simulink subsystem "ApplFOCSLLowPrio"  (R2024b)
settings: Solver=VariableStepAuto  StartTime=0.0  StopTime=10.0  RelTol=1e-3
undefined symbols (not defined in the file or in its folder): inverter, pmsm, PU_System
libraries: slpidlib x1
settings Model: Creator=The MathWorks, Inc.  LastModifiedBy=snarayan
settings RTWCC: GPUComputeCapability=3.5  LargeConstantGeneration=WriteOnlyDNNConstantsToDataFiles

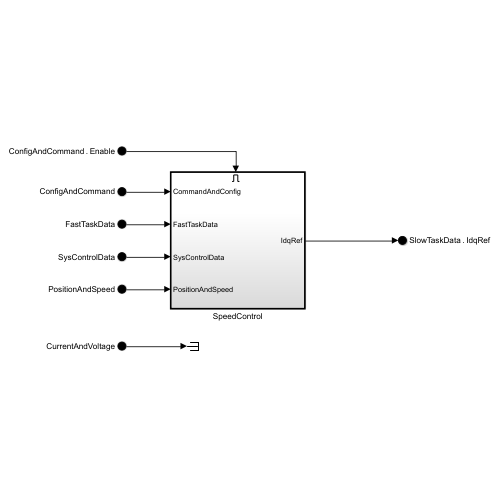
[thumbnail: Simulink's stored preview of the top-level diagram]
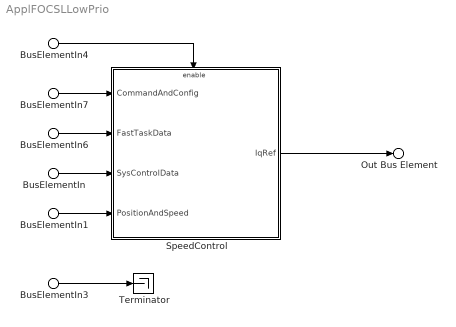
== system ApplFOCSLLowPrio ==
  BusElementIn7 : Inport  PortName=ConfigAndCommand
  BusElementIn4 : Inport  PortName=ConfigAndCommand  Element=Enable
  BusElementIn3 : Inport  Port=2  PortName=CurrentAndVoltage
  BusElementIn1 : Inport  Port=3  PortName=PositionAndSpeed
  BusElementIn6 : Inport  Port=4  PortName=FastTaskData
  BusElementIn : Inport  Port=5  PortName=SysControlData
  SpeedControl : Subsystem
  Terminator : Terminator
  Out Bus Element : Outport  PortName=SlowTaskData  Element=IqRef
  wires:
  BusElementIn4/1 -> SpeedControl/Enable
  SpeedControl/1(IqRef) -> Out Bus Element/1
  BusElementIn7/1 -> SpeedControl/1(CommandAndConfig)
  BusElementIn6/1 -> SpeedControl/2(FastTaskData)
  BusElementIn/1 -> SpeedControl/3(SysControlData)
  BusElementIn1/1 -> SpeedControl/4(PositionAndSpeed)
  BusElementIn3/1 -> Terminator/1

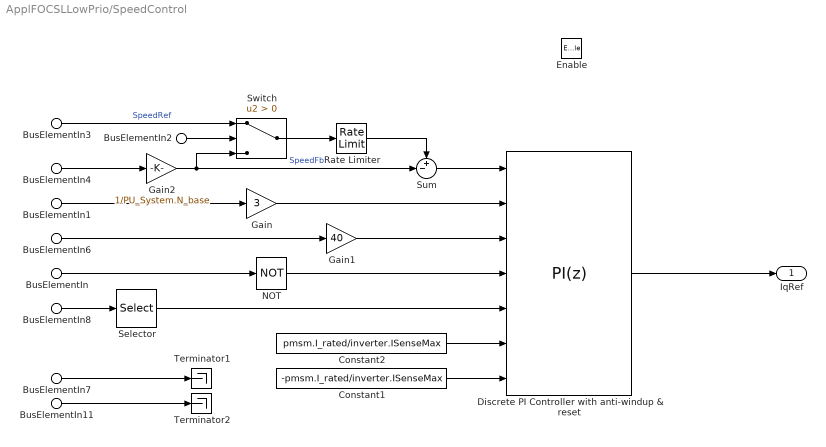
== system ApplFOCSLLowPrio/SpeedControl ==
  BusElementIn11 : Inport  PortName=CommandAndConfig
  BusElementIn : Inport  Port=2  PortName=FastTaskData  Element=EnClosedLoop
  BusElementIn2 : Inport  Port=2  PortName=FastTaskData  Element=EnClosedLoop
  BusElementIn4 : Inport  Port=2  PortName=FastTaskData  Element=Speed
  BusElementIn8 : Inport  Port=2  PortName=FastTaskData  Element=Idq
  BusElementIn1 : Inport  Port=3  PortName=SysControlData  Element=PIGains.Speed_Kp
  BusElementIn6 : Inport  Port=3  PortName=SysControlData  Element=PIGains.Speed_Ki*Tsc
  BusElementIn3 : Inport  Port=3  PortName=SysControlData  Element=SpeedRef
  BusElementIn7 : Inport  Port=4  PortName=PositionAndSpeed
  Enable : EnablePort
  Constant1 : Constant  Value=-pmsm.I_rated/inverter.ISenseMax  OutDataTypeStr=dataType
  Constant2 : Constant  Value=pmsm.I_rated/inverter.ISenseMax  OutDataTypeStr=dataType
  Discrete PI Controller with anti-windup & reset : slpidlib/PID Controller  Controller=PI  Form=Parallel  TimeDomain=Discrete-time  UseExternalTs=off  SampleTime=-1  IntegratorMethod=Forward Euler  FilterMethod=Forward Euler  ControllerParametersSource=external  P=1  I=1  UseKiTs=on  D=0  UseExternalDerivativeSource=off  N=100  UseFilter=on  TunerSelectOption=Transfer Function Based (PID Tuner App)  InitialConditionSource=external  InitialConditionForIntegrator=0  InitialConditionForFilter=0  DifferentiatorICPrevScaledInput=0  ExternalReset=level  TrackingMode=off  Kt=1  LimitOutput=on  SatLimitsSource=external  UpperSaturationLimit=1  LowerSaturationLimit=-1  LinearizeAsGain=on  AntiWindupMode=clamping  Kb=1  LimitIntegrator=off  UpperIntegratorSaturationLimit=inf  LowerIntegratorSaturationLimit=-inf  RndMeth=Simplest  POutMin=[]  POutMax=[]  IOutMin=[]  IOutMax=[]  DOutMin=[]  DOutMax=[]  NOutMin=[]  NOutMax=[]  SumOutMin=[]  SumOutMax=[]  SaturationOutDataTypeStr=Inherit: Inherit via back propagation  SaturationOutMin=[]  SaturationOutMax=[]  PParamMin=[]  PParamMax=[]  IParamMin=[]  IParamMax=[]  DParamMin=[]  DParamMax=[]  NParamMin=[]  NParamMax=[]  KbParamMin=[]  KbParamMax=[]  KtParamMin=[]  KtParamMax=[]  KbOutMin=[]  KbOutMax=[]  KtOutMin=[]  KtOutMax=[]  IntegratorOutMin=[]  IntegratorOutMax=[]  FilterOutMin=[]  FilterOutMax=[]  SumI1OutMin=[]  SumI1OutMax=[]  SumI2OutMin=[]  SumI2OutMax=[]  SumI3OutMin=[]  SumI3OutMax=[]  SumI4OutMin=[]  SumI4OutMax=[]  SumDOutMin=[]  SumDOutMax=[]  DifferentiatorOutMin=[]  DifferentiatorOutMax=[]  FilterDiffOutCoefMin=[]  FilterDiffOutCoefMax=[]  ReciprocalOutMin=[]  ReciprocalOutMax=[]  SumDenOutMin=[]  SumDenOutMax=[]  SumNumOutMin=[]  SumNumOutMax=[]  DivideOutMin=[]  DivideOutMax=[]  UdiffTsProdOutMin=[]  UdiffTsProdOutMax=[]  NTsProdOutMin=[]  NTsProdOutMax=[]  UintegralTsProdOutMin=[]  UintegralTsProdOutMax=[]  UngainTsProdOutMin=[]  UngainTsProdOutMax=[]  ClampingZeroOutDataTypeStr=Inherit: Inherit via back propagation  ClampingZeroOutMin=[]  ClampingZeroOutMax=[]  FilterDenConstantOutDataTypeStr=Inherit: Inherit via back propagation  FilterDenConstantOutMin=[]  FilterDenConstantOutMax=[]  PCopyOutDataTypeStr=Inherit: Inherit via back propagation  PCopyOutMin=[]  PCopyOutMax=[]  NCopyOutDataTypeStr=Inherit: Inherit via back propagation  NCopyOutMin=[]  NCopyOutMax=[]  IntegratorContinuousStateAttributes=''  IntegratorStateMustResolveToSignalObject=off  IntegratorRTWStateStorageClass=Auto  FilterContinuousStateAttributes=''  FilterStateMustResolveToSignalObject=off  FilterRTWStateStorageClass=Auto  ParallelPVariant=ExternalParameters  IdealPVariant=Disabled  IVariant=ExternalParameters  DVariant=Disabled  IntegratorVariant=Discrete  SatVariant=External  AWVariant=DiscClampingParallel  PCopyVariant=Disabled  TRVariant=Disabled  FdbkBlocksVariant=Forward  IdealPFdbkVariant=Disabled  SatFdbkVariant=Disabled  DerivativeFilterVariant=Disabled  NVariant=Disabled  NCopyVariant=Disabled_SignalSpec  FilterICVariant=Disabled  IntegratorICVariant=ExternalICs  ExternalResetVariant=ExternalReset  TRSumVariant=Passthrough  SumFdbkVariant=Disabled  SumVariant=Sum_PI  TsampFilterVariant=InternalTs  TsampNgainVariant=Passthrough  TsampIntegralVariant=Disabled_SignalSpec  ExternalSaturationOutDataTypeStr=Inherit: Same as second input  DerivativeSourceVariant=Disabled  PreIntVariant=InternalPreInt
  Gain : Gain  Gain=3  RndMeth=Simplest  OutDataTypeStr=Inherit: Same as input
  Gain1 : Gain  Gain=40  RndMeth=Simplest  OutDataTypeStr=Inherit: Same as input
  Gain2 : Gain  Gain=1/PU_System.N_base  RndMeth=Simplest  OutDataTypeStr=Inherit: Same as input
  NOT : Logic  Operator=NOT  IconShape=distinctive  AllPortsSameDT=off  OutDataTypeStr=boolean
  Rate Limiter : RateLimiter  RisingSlewLimit=0.2  FallingSlewLimit=-0.2  SampleTimeMode=inherited
  Selector : Selector  InputPortWidth=2  IndexOptions=Index vector (dialog)  Indices=[2]  OutputSizes=1
  Sum : Sum  Inputs=+-|  OutDataTypeStr=Inherit: Same as first input
  Switch : Switch  Criteria=u2 > Threshold  SaturateOnIntegerOverflow=off  InputSameDT=off
  Terminator1 : Terminator
  Terminator2 : Terminator
  IqRef : Outport
  wires:
  Gain1/1 -> Discrete PI Controller with anti-windup & reset/3
  Gain/1 -> Discrete PI Controller with anti-windup & reset/2
  BusElementIn6/1 -> Gain1/1
  BusElementIn1/1 -> Gain/1
  BusElementIn2/1 -> Switch/2
  Rate Limiter/1 -> Sum/1
  NOT/1 -> Discrete PI Controller with anti-windup & reset/4
  Selector/1 -> Discrete PI Controller with anti-windup & reset/5
  BusElementIn4/1 -> Gain2/1
  BusElementIn8/1 -> Selector/1
  Gain2/1 -> Sum/2, Switch/3  "SpeedFb"
  Discrete PI Controller with anti-windup & reset/1 -> IqRef/1
  BusElementIn11/1 -> Terminator2/1
  BusElementIn3/1 -> Switch/1  "SpeedRef"
  Constant1/1 -> Discrete PI Controller with anti-windup & reset/7
  Constant2/1 -> Discrete PI Controller with anti-windup & reset/6
  BusElementIn7/1 -> Terminator1/1
  Switch/1 -> Rate Limiter/1
  BusElementIn/1 -> NOT/1
  Sum/1 -> Discrete PI Controller with anti-windup & reset/1
